simulink model "testing1"  (R2023b)
settings: Solver=ode4  StartTime=0.0  StopTime=inf  FixedStep=0.01  RelTol=1e-3  EnableMultiTasking=on
undefined symbols (not defined in the file): DiscIntNeverNeededParam
libraries: stm32f4xxblockslib x7, simulink x4, stm32l4xxblockslib x4
settings Model: STM32="{\"AnalogInput\":[{\"ID\":\"untitled1:22\"},{\"ID\":\"testing:106\"},{\"ID\":\"testing1:106\"}],\"DigitalPortWrite\":[{\"ID\":\"untitled1:41\"},{\"ID\":\"untitled1:58\"},{\"ID\":\"testing:125\"},{\"ID\":\"testing:142\"},{\"ID\":\"testing1:125\"},{\"ID\":\"testing1:142\"}],\"PWMOutput\":[{\"ID\":\"untitled1:43\"},{\"ID\":\"untitled1:60\"},{\"ID\":\"testing:127\"},{\"ID\":\"testing:144\"},{\"ID\":\"testing1:127\"},{\"ID\":\"testing1:144\"}],\"DigitalPortRead\":[{\"ID\":\"untitled1:49\"},{\"ID\":\"untitled1:50\"},{\"ID\":\"untitled1:67\"},{\"ID\":\"untitled1:68\"},{\"ID\":\"testing:133\"},{\"ID\":\"testing:134\"},{\"ID\":\"testing:151\"},{\"ID\":\"testing:152\"},{\"ID\":\"testing1:133\"},{\"ID\":\"testing1:134\"},{\"ID\":\"testing1:151\"},{\"ID\":\"testing1:152\"}],\"HardwareInterrupt\":[{\"ID\":\"testing:124\"},{\"ID\":\"testing:141\"},{\"ID\":\"testing1:124\"},{\"ID\":\"testing1:141\"}]}"  Creator=ofekn  LastModifiedBy=ofekn
settings SolverCC: AutoInsertRateTranBlk=on
settings OptimizationCC: DefaultParameterBehavior=Inlined  EnhancedBackFolding=on  PassReuseOutputArgsAs=Individual arguments  ZeroExternalMemoryAtStartup=off  ZeroInternalMemoryAtStartup=off  MaxStackSize=512  OptimizeBlockOrder=speed  DifferentSizesBufferReuse=on  OptimizationCustomize=off  EfficientTunableParamExpr=on
settings DebuggingCC: ParameterTunabilityLossMsg=error
settings HardwareCC: ProdBitPerPointer=32  ProdBitPerSizeT=32  ProdBitPerPtrDiffT=32  ProdLargestAtomicInteger=Long  ProdLargestAtomicFloat=Double  ProdWordSize=32  ProdLongLongMode=on  ProdHWDeviceType=ARM Compatible->ARM Cortex-M
settings SFSimCC: MATLABDynamicMemAlloc=off
settings RTWCC: Description=Embedded Coder  SystemTargetFile=ert.tlc  HardwareBoard=STM32L4xx Based  TemplateMakefile=ert_default_tmf  Toolchain=GNU Tools for ARM Embedded Processors  GPUComputeCapability=5.0
settings CodeAppCC: ForceParamTrailComments=on  IgnoreCustomStorageClasses=off  OperatorAnnotations=on  SimulinkDataObjDesc=on  SFDataObjDesc=on  InsertBlockDesc=on
settings ERTTargetCC: TargetLangStandard=C99 (ISO)  CodeReplacementLibrary=ARM Cortex-M  ExtModeTransport=3  ExtModeStaticAlloc=on  ExtModeStaticAllocSize=2048  ExtModeMexFile=ext_xcp  ExtModeIntrfLevel=Level2 - Open  InlinedParameterPlacement=NonHierarchical
settings SettingsController: UseSoCProfilerForTargets=0

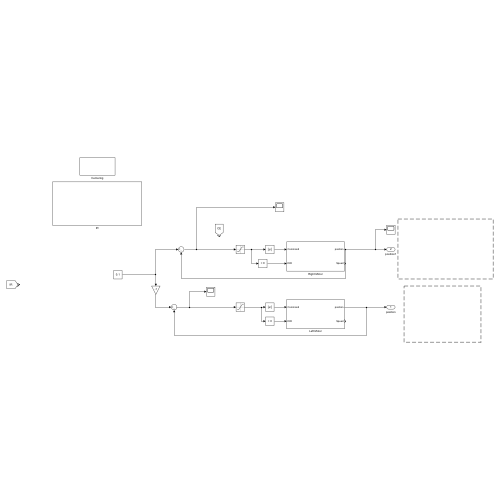
[thumbnail: Simulink's stored preview of the top-level diagram]
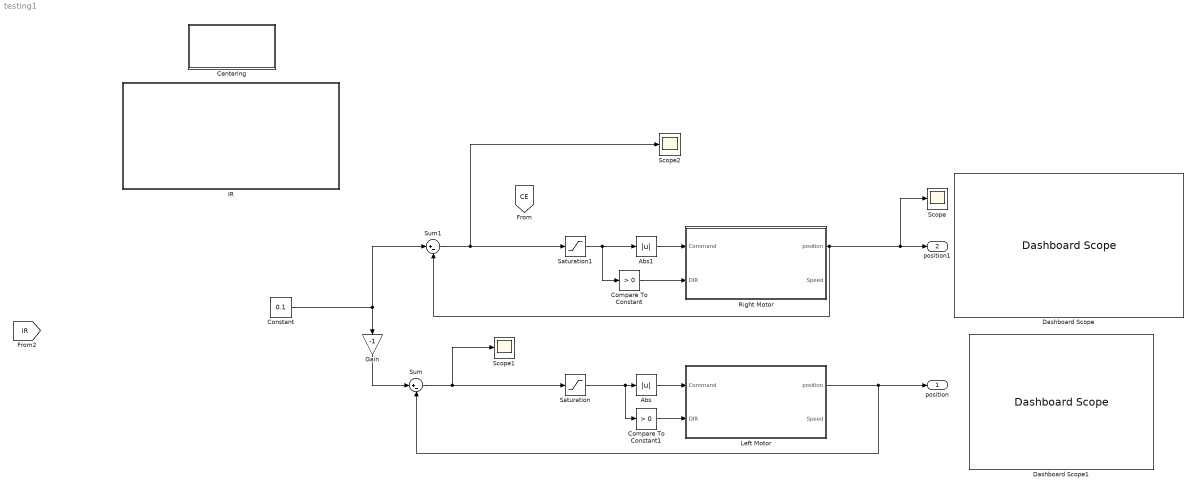
== system testing1 ==
  Abs : Abs  SaturateOnIntegerOverflow=off
  Abs1 : Abs  SaturateOnIntegerOverflow=off
  Centering : Subsystem
  Compare To Constant : simulink/Logic and Bit Operations/Compare To Constant  relop=>  const=0  OutDataTypeStr=boolean
  Compare To Constant1 : simulink/Logic and Bit Operations/Compare To Constant  relop=>  const=0  OutDataTypeStr=boolean
  Constant : Constant  Value=0.1
  Dashboard Scope : DashboardScope
  Dashboard Scope1 : DashboardScope
  Gain : Gain  Gain=-1
  IR : Subsystem
  Left Motor : Subsystem
  Right Motor : Subsystem
  Saturation : Saturate  UpperLimit=99  LowerLimit=-99
  Saturation1 : Saturate  UpperLimit=99  LowerLimit=-99
  Scope : Scope
  Scope1 : Scope
  Scope2 : Scope
  Sum : Sum  Inputs=|+-
  Sum1 : Sum  Inputs=|+-
  position : Outport
  position1 : Outport  Port=2
  wires:
  Right Motor/1(position) -> Sum1/2, Scope/1, position1/1
  Sum/1 -> Saturation/1, Scope1/1
  Left Motor/1(position) -> position/1, Sum/2
  Constant/1 -> Gain/1, Sum1/1
  Saturation1/1 -> Abs1/1, Compare To Constant/1
  Abs1/1 -> Right Motor/1(Command)
  Saturation/1 -> Compare To Constant1/1, Abs/1
  Compare To Constant1/1 -> Left Motor/2(DIR)
  Abs/1 -> Left Motor/1(Command)
  Compare To Constant/1 -> Right Motor/2(DIR)
  Sum1/1 -> Saturation1/1, Scope2/1
  Gain/1 -> Sum/1

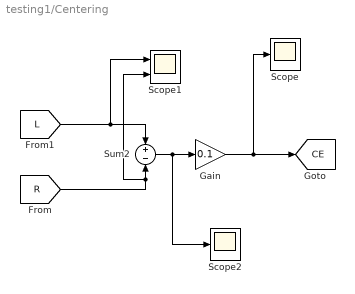
== system testing1/Centering ==
  Gain : Gain  Gain=0.1
  Scope : Scope
  Scope1 : Scope  NumInputPorts=2
  Scope2 : Scope
  Sum2 : Sum  Inputs=+|-
  tag scope: CE=global
  wires:
  [R] -> Scope1/2, Sum2/2
  [L] -> Scope1/1, Sum2/1
  Sum2/1 -> Scope2/1, Gain/1
  Gain/1 -> Scope/1, [CE]

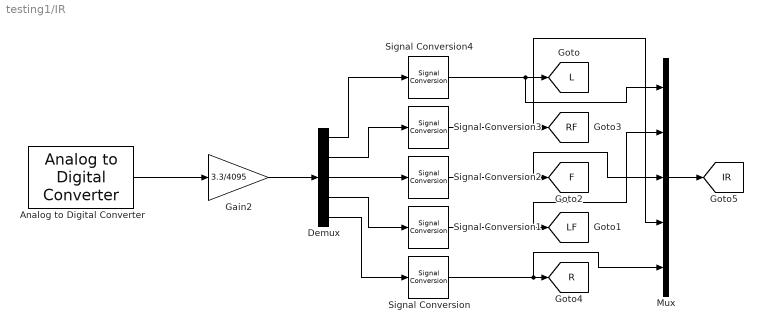
== system testing1/IR ==
  Analog to Digital Converter : stm32f4xxblockslib/Analog to Digital Converter  ADCModule=ADC1  ConversionGroup=Regular  TriggerMode=Trigger and read  NumberOfConversions=5  EnableBufferConv=off  BufferLength=1  OutputStatus=off  SampleTime=-1  EnableSimPort=off  hoistedMaskSrc=ECSoC/ECSimCodegen/Analog to Digital Converter
      settings: LibrarySourceBlock=stm32l4xxblockslib/Analog to Digital Converter
  Demux : Demux  Outputs=5
  Gain2 : Gain  Gain=3.3/4095
  Mux : Mux  Inputs=5
  Signal Conversion{,1..4} (5 alike) : SignalConversion  OverrideOpt=off
  tag scope: F=global, IR=global, L=global, LF=global, R=global, RF=global
  wires:
  Demux/3 -> Signal Conversion2/1
  Demux/5 -> Signal Conversion/1
  Demux/4 -> Signal Conversion1/1
  Signal Conversion3/1 -> Mux/4, [RF]
  Analog to Digital Converter/1 -> Gain2/1
  Gain2/1 -> Demux/1
  Demux/2 -> Signal Conversion3/1
  Demux/1 -> Signal Conversion4/1
  Signal Conversion2/1 -> Mux/3, [F]
  Signal Conversion/1 -> Mux/5, [R]
  Signal Conversion1/1 -> Mux/2, [LF]
  Signal Conversion4/1 -> Mux/1, [L]
  Mux/1 -> [IR]

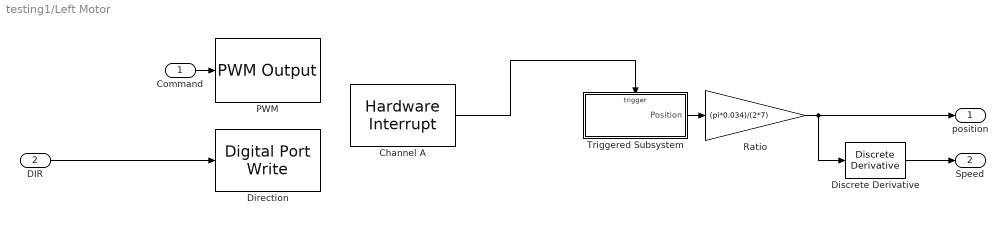
== system testing1/Left Motor ==
  Command : Inport
  DIR : Inport  Port=2
  Channel A : stm32l4xxblockslib/Hardware Interrupt  ISRGroup=External interrupts (EXTI)  ISRName=EXTI3_IRQHandler  ISRNumber=24  EventsList={ 'on', 'EXTI3 Event', '1'; 'off', 'Custom event', '2' }  SelectedEvents={'EXTI3 Event'}  TaskPriority=30  DisablePreemption=off  ClearInterruptFlagsAtEndOfEvent=off  InterruptDefinitionFile=$(TARGET_ROOT)/registry/interrupts/STM32F4xxBased_interrupts.xml  HardwareBoard=STM32L4xx Based  EnableSimPort=off
  Direction : stm32f4xxblockslib/Digital Port Write  PortName=GPIOA  PinNumber=[12]  ReadOperation=off  IOAsArray=on  EnableSimPort=off  hoistedMaskSrc=ECSoC/ECSimCodegen/Digital Port Write
      settings: LibrarySourceBlock=stm32l4xxblockslib/Digital Port Write
  Discrete Derivative : simulink/Discrete/Discrete Derivative  gainval=1.0  ICPrevScaledInput=0.0  OutMin=[]  OutMax=[]  OutDataType=fixdt(1, 16)  OutScaling=2^-10  DoSatur=off
  PWM : stm32l4xxblockslib/PWM Output  TimerModule=TIM16  DutycycleUnits=Percentage  EnableChannel1=on  EnableChannel2=off  EnableChannel3=off  EnableChannel4=off  EnableChannel5=off  EnableChannel6=off  EnableCounterInput=off  EnableMainOutputInput=off  EnableFrequencyInput=off  SetRCAfterCE=off  OutputDirection=off  OutputMainOutputEnableStatus=off  SampleTime=0.1  EnableSimPort=off  EnableUpdateEvent=off  EnableCaptureCompare1Event=off  EnableCaptureCompare2Event=off  EnableCaptureCompare3Event=off  EnableCaptureCompare4Event=off  EnableTriggerEvent=off  EnableBreakEvent=off  EnableBreakEvent2=off  ProcessorFamily=STM32L4  hoistedMaskSrc=ECSoC/ECSimCodegen/PWM Output
  Ratio : Gain  Gain=(pi*0.034)/(2*7)
  Triggered Subsystem : Subsystem  TreatAsAtomicUnit=on
  position : Outport
  Speed : Outport  Port=2
  wires:
  Command/1 -> PWM/1
  Triggered Subsystem/1(Position) -> Ratio/1
  Channel A/1 -> Triggered Subsystem/Trigger
  Discrete Derivative/1 -> Speed/1
  Ratio/1 -> position/1, Discrete Derivative/1
  DIR/1 -> Direction/1

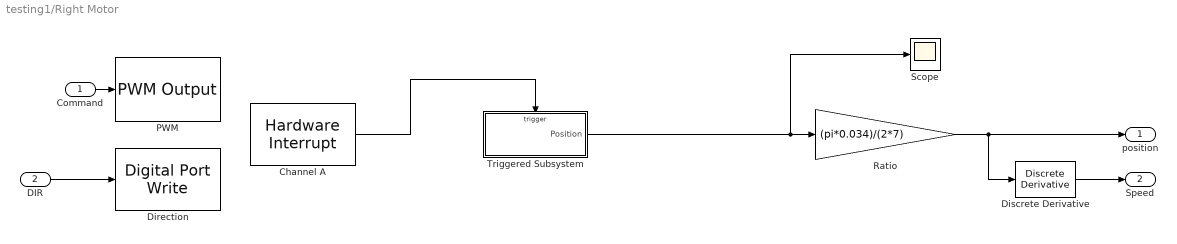
== system testing1/Right Motor ==
  Command : Inport
  DIR : Inport  Port=2
  Channel A : stm32l4xxblockslib/Hardware Interrupt  ISRGroup=External interrupts (EXTI)  ISRName=EXTI0_IRQHandler  ISRNumber=21  EventsList={ 'on', 'EXTI0 Event', '1'; 'off', 'Custom event', '2' }  SelectedEvents={'EXTI0 Event'}  TaskPriority=30  DisablePreemption=off  ClearInterruptFlagsAtEndOfEvent=off  InterruptDefinitionFile=$(TARGET_ROOT)/registry/interrupts/STM32F4xxBased_interrupts.xml  HardwareBoard=STM32L4xx Based  EnableSimPort=off
  Direction : stm32f4xxblockslib/Digital Port Write  PortName=GPIOA  PinNumber=[11]  ReadOperation=off  IOAsArray=on  EnableSimPort=off  hoistedMaskSrc=ECSoC/ECSimCodegen/Digital Port Write
      settings: LibrarySourceBlock=stm32l4xxblockslib/Digital Port Write
  Discrete Derivative : simulink/Discrete/Discrete Derivative  gainval=1.0  ICPrevScaledInput=0.0  OutMin=[]  OutMax=[]  OutDataType=fixdt(1, 16)  OutScaling=2^-10  DoSatur=off
  PWM : stm32l4xxblockslib/PWM Output  TimerModule=TIM1  DutycycleUnits=Percentage  EnableChannel1=on  EnableChannel2=off  EnableChannel3=off  EnableChannel4=off  EnableChannel5=off  EnableChannel6=off  EnableCounterInput=off  EnableMainOutputInput=off  EnableFrequencyInput=off  SetRCAfterCE=off  OutputDirection=off  OutputMainOutputEnableStatus=off  SampleTime=0.1  EnableSimPort=off  EnableUpdateEvent=off  EnableCaptureCompare1Event=off  EnableCaptureCompare2Event=off  EnableCaptureCompare3Event=off  EnableCaptureCompare4Event=off  EnableTriggerEvent=off  EnableBreakEvent=off  EnableBreakEvent2=off  ProcessorFamily=STM32L4  hoistedMaskSrc=ECSoC/ECSimCodegen/PWM Output
  Ratio : Gain  Gain=(pi*0.034)/(2*7)
  Scope : Scope
  Triggered Subsystem : Subsystem  TreatAsAtomicUnit=on
  position : Outport
  Speed : Outport  Port=2
  wires:
  Command/1 -> PWM/1
  Channel A/1 -> Triggered Subsystem/Trigger
  Discrete Derivative/1 -> Speed/1
  Ratio/1 -> position/1, Discrete Derivative/1
  Triggered Subsystem/1(Position) -> Scope/1, Ratio/1
  DIR/1 -> Direction/1

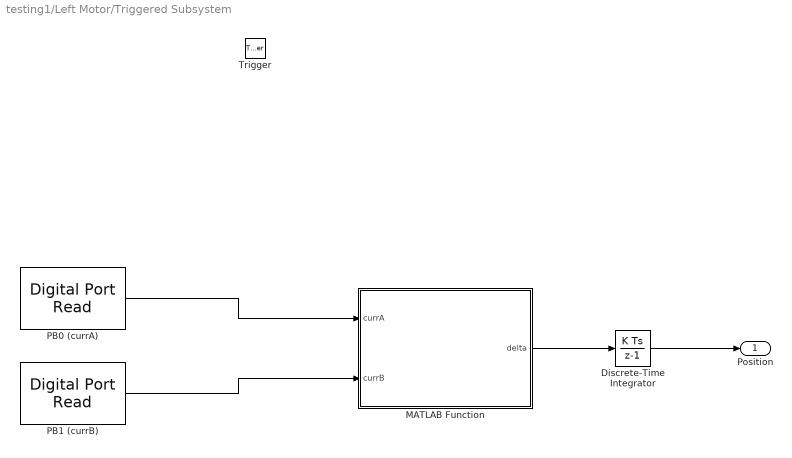
== system testing1/Left Motor/Triggered Subsystem ==
  Trigger : TriggerPort  TriggerType=function-call  VariantControl=(inherit)
  Discrete-Time Integrator : DiscreteIntegrator  SampleTime=-1  ICPrevOutput=DiscIntNeverNeededParam  ICPrevScaledInput=DiscIntNeverNeededParam
  MATLAB Function : MATLAB Function  TreatAsAtomicUnit=on
  PB0 (currA) : stm32f4xxblockslib/Digital Port Read  PortName=GPIOB  PinNumber=[3]  ReadOperation=on  IOAsArray=on  SampleTime=-1  EnableSimPort=off  hoistedMaskSrc=ECSoC/ECSimCodegen/Digital Port Read
      settings: LibrarySourceBlock=stm32l4xxblockslib/Digital Port Read
  PB1 (currB) : stm32f4xxblockslib/Digital Port Read  PortName=GPIOB  PinNumber=[4]  ReadOperation=on  IOAsArray=on  SampleTime=-1  EnableSimPort=off  hoistedMaskSrc=ECSoC/ECSimCodegen/Digital Port Read
      settings: LibrarySourceBlock=stm32l4xxblockslib/Digital Port Read
  Position : Outport
  wires:
  PB1 (currB)/1 -> MATLAB Function/2(currB)
  PB0 (currA)/1 -> MATLAB Function/1(currA)
  Discrete-Time Integrator/1 -> Position/1
  MATLAB Function/1(delta) -> Discrete-Time Integrator/1

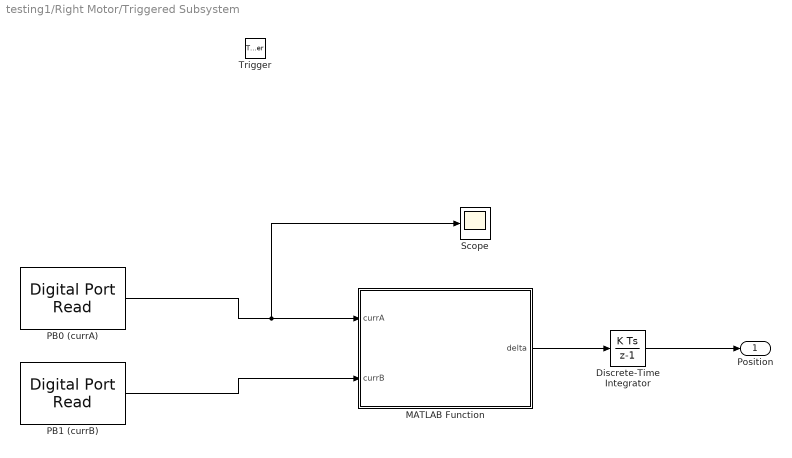
== system testing1/Right Motor/Triggered Subsystem ==
  Trigger : TriggerPort  TriggerType=function-call  VariantControl=(inherit)
  Discrete-Time Integrator : DiscreteIntegrator  SampleTime=-1  ICPrevOutput=DiscIntNeverNeededParam  ICPrevScaledInput=DiscIntNeverNeededParam
  MATLAB Function : MATLAB Function  TreatAsAtomicUnit=on
  PB0 (currA) : stm32f4xxblockslib/Digital Port Read  PortName=GPIOB  PinNumber=[0]  ReadOperation=on  IOAsArray=on  SampleTime=-1  EnableSimPort=off  hoistedMaskSrc=ECSoC/ECSimCodegen/Digital Port Read
      settings: LibrarySourceBlock=stm32l4xxblockslib/Digital Port Read
  PB1 (currB) : stm32f4xxblockslib/Digital Port Read  PortName=GPIOB  PinNumber=[1]  ReadOperation=on  IOAsArray=on  SampleTime=-1  EnableSimPort=off  hoistedMaskSrc=ECSoC/ECSimCodegen/Digital Port Read
      settings: LibrarySourceBlock=stm32l4xxblockslib/Digital Port Read
  Scope : Scope
  Position : Outport
  wires:
  PB1 (currB)/1 -> MATLAB Function/2(currB)
  PB0 (currA)/1 -> Scope/1, MATLAB Function/1(currA)
  MATLAB Function/1(delta) -> Discrete-Time Integrator/1
  Discrete-Time Integrator/1 -> Position/1

== matlab function testing1/Left Motor/Triggered Subsystem/MATLAB Function ==
  data: delta output; currA input; currB input
function delta = decodeSimple(currA, currB)
    if (currA == currB)
        delta = +1;   % Forward
    else
        delta = -1;   % Reverse
    end
end

== matlab function testing1/Right Motor/Triggered Subsystem/MATLAB Function ==
  data: delta output; currA input; currB input
function delta = decodeSimple(currA, currB)
    if (currA == currB)
        delta = -1;   % Forward
    else
        delta = +1;   % Reverse
    end
end
